simulink model "Formation"  (R2024b)
settings: Solver=ode4  StartTime=0.0  StopTime=50  RelTol=1e-3
libraries: simulink x5
settings Model: Creator=Omar  LastModifiedBy=Omar

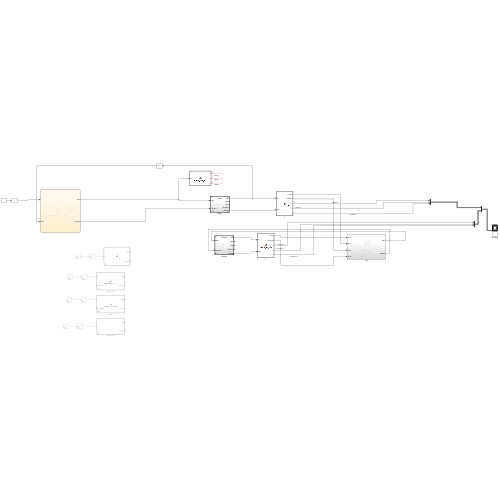
[thumbnail: Simulink's stored preview of the top-level diagram]
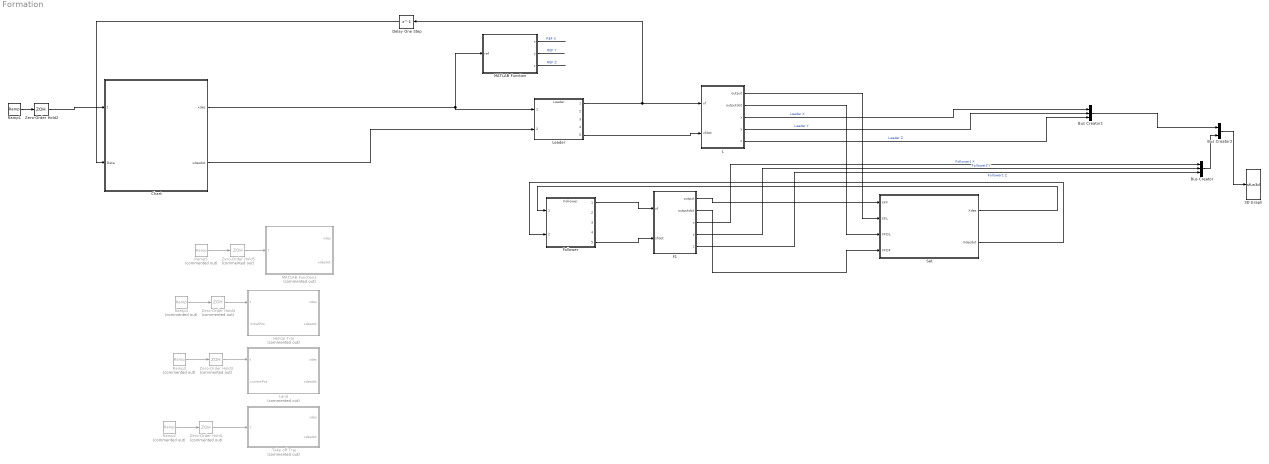
== system Formation ==
  3D Graph : S-Function  LoadFcn=if exist('sfun3d','file'), sfun3d([],[],[],'LoadBlock'); end  FunctionName=sfun3d  Parameters=ax,T,np,cp,gd,ls,mk,mx,hd,tb  SFunctionDeploymentMode=off  EnableBusSupport=off  mask(3D Graph){np=2, ax=[-2 2 -2 2 0 10], mx=1e4, T=0.1, cp=[2 1 3], gd=on, hd=on, tb=off, ls=-, mk=none}
      mask prompts: np "Number of moving points (lines)"; ax "Range: [xmin xmax  ymin ymax zmin zmax]"; mx "Max number of points in each line"; T "Sampling Time"; cp "Camera position (use [0 0 1] for 2D XY view)"; gd "Grid (on|off)"; hd "HeadMarkers (on|off)"; tb "Toolbar (on|off)"; ls "LineStyle"; mk "LineMarker"
      mask help:
      | This block plots the position of several points in the XYZ space. The input contains the coordinates of all the points (x1,y1,z1,x2,y2,z2,...).
      | The number of moving points (lines), the XYZ ranges, sampling time, camera position, and grid (among other things) can be set as mask parameters.
      settings: CopyFcn=if exist('sfun3d','file'), sfun3d([],[],[],'CopyBlock'); end  DeleteFcn=if exist('sfun3d','file'), sfun3d([],[],[],'DeleteBlock'); end  NameChangeFcn=if exist('sfun3d','file'), sfun3d([],[],[],'NameChange'); end
      mask Help:
      | This block plots the position of several points in the XYZ space. The input contains the coordinates of all the points (x1,y1,z1,x2,y2,z2,...).
      | The number of moving points (lines), the XYZ ranges, sampling time, camera position, and grid (among other things) can be set as mask parameters.
      mask TypeOptions ls: - | -- | : | -. | none
      mask TypeOptions mk: none | . | + | o | * | x | square | diamond | v | ^ | > | < | pentagram | hexagram
      mask Display: plot([.05 .95 .95 .05 .05],[.45 .45 .95 .95 .45], 0.5+cos(0:0.1:2*pi)*0.3,0.7+sin(0:0.1:2*pi)*0.2)
  Bus Creator : BusCreator  Inputs=3
  Bus Creator1 : BusCreator  Inputs=3
  Bus Creator2 : BusCreator  Inputs=2
  Chart : Stateflow chart  TreatAsAtomicUnit=on
      settings: PortSchema="{\"entries\":[{\"content\":{\"sides\":[{\"content\":{\"connectorIds\":[\"In1\",\"In2\"]},\"type\":\"ConnectorPlacement.EquallySpacedRectSide\",\"uuid\":\"b3e650a5-816a-4038-bd6f-7a09548ffccf\"},{\"content\":{\"connectorIds\":[\"Out2\",\"Out1\"],\"side\":\"RIGHT\"},\"type\":\"ConnectorPlacement.EquallySpacedRectSide\",\"uuid\":\"881456fa-c96c-4b3e-8437-ce6d3f72eb13\"},{\"content\":{\"side\":\"TOP\"},\"type\":\"ConnectorPlacement.EquallySpacedRectSide\",\"uuid\":\"2026285f-4a20-43d0-8312-bd14694b0db2\"}]},\"type\":\"ConnectorPlacement.EquallySpacedConnector\",\"uuid\":\"eb1cc1af-b444-4b44-9b14-5798d5451655\"}],\"packageUris\":[\"http://schema.mathworks.com/mf0/Connector/R2020b\"],\"version\":\"1.0\"}"
  Delay One Step : Delay  DelayLength=1
  F1 : MATLAB Function  TreatAsAtomicUnit=on
  Follower : ModelReference  ModelNameDialog=Follower.slx  SimulationMode=Normal  ModelReferenceVersion=10.12
  Helical Traj : MATLAB Function  Commented=on  TreatAsAtomicUnit=on
  L : MATLAB Function  TreatAsAtomicUnit=on
  Land : MATLAB Function  Commented=on  TreatAsAtomicUnit=on
  Leader : ModelReference  ModelNameDialog=Leader.slx  SimulationMode=Normal  ModelReferenceVersion=10.10
  MATLAB Function : MATLAB Function  TreatAsAtomicUnit=on
  MATLAB Function1 : MATLAB Function  Commented=on  TreatAsAtomicUnit=on
  Ramp1 : simulink/Sources/Ramp  slope=1  start=0  InitialOutput=0
  Ramp{2..5} (4 alike) : simulink/Sources/Ramp  Commented=on  slope=1  start=0  InitialOutput=0
  Sat : Subsystem
  Take off Traj : MATLAB Function  Commented=on  TreatAsAtomicUnit=on
  Zero-Order Hold{1,3..5} (4 alike) : ZeroOrderHold  Commented=on  SampleTime=0.02
  Zero-Order Hold2 : ZeroOrderHold  SampleTime=0.02
  wires:
  L/3(x) -> Bus Creator1/1  "Leader X"
  L/4(y) -> Bus Creator1/2  "Leader Y"
  L/5(z) -> Bus Creator1/3  "Leader Z"
  F1/4(y) -> Bus Creator/2  "Follower1 Y"
  F1/5(z) -> Bus Creator/3  "Follower1 Z"
  Follower/1 -> F1/1(xf)
  F1/3(x) -> Bus Creator/1  "Follower1 X"
  MATLAB Function/2(y) -> ?  "REF Y"
  MATLAB Function/3(z) -> ?  "REF Z"
  MATLAB Function/1(x) -> ?  "REF X"
  Leader/5 -> L/2(xfdot)
  Follower/5 -> F1/2(xfdot)
  Bus Creator2/1 -> 3D Graph/1
  Bus Creator1/1 -> Bus Creator2/1
  Bus Creator/1 -> Bus Creator2/2
  L/2(outputdot) -> Sat/3(XFDL)
  L/1(output) -> Sat/2(XFL)
  Ramp1/1 -> Zero-Order Hold2/1
  Ramp2/1 -> Zero-Order Hold1/1
  Zero-Order Hold1/1 -> Take off Traj/1(t)
  Ramp3/1 -> Zero-Order Hold3/1
  Zero-Order Hold3/1 -> Land/1(t)
  Zero-Order Hold4/1 -> Helical Traj/1(t)
  Ramp4/1 -> Zero-Order Hold4/1
  Zero-Order Hold2/1 -> Chart/1(t)
  Leader/1 -> Delay One Step/1, L/1(xf)
  Delay One Step/1 -> Chart/2(Data)
  F1/2(outputdot) -> Sat/4(XFDF)
  F1/1(output) -> Sat/1(XFF)
  Ramp5/1 -> Zero-Order Hold5/1
  Zero-Order Hold5/1 -> MATLAB Function1/1(t)
  Chart/2(xdes) -> Leader/1, MATLAB Function/1(ref)
  Chart/1(xdesdot) -> Leader/2
  Sat/2(Xdesdot) -> Follower/2
  Sat/1(Xdes) -> Follower/1

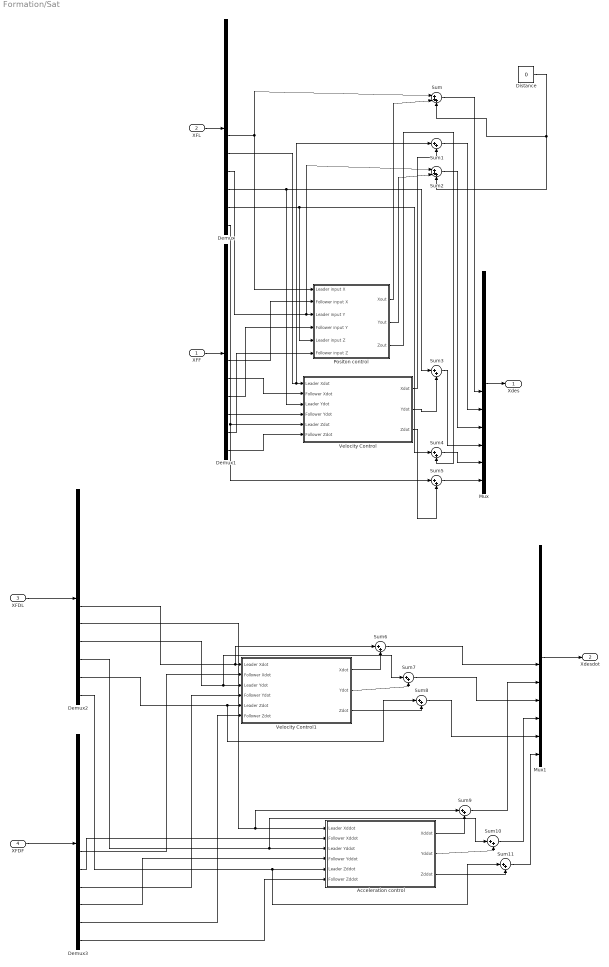
== system Formation/Sat ==
  XFF : Inport
  XFL : Inport  Port=2
  XFDL : Inport  Port=3
  XFDF : Inport  Port=4
  Acceleration control : Subsystem
  Demux{,1..3} (4 alike) : Demux  Outputs=12
  Distance : Constant  Value=0
  Mux : Mux  Inputs=12
  Mux1 : Mux  Inputs=12
  Positon control : Subsystem
  Sum : Sum  Inputs=|+++
  Sum{1,3..11} (10 alike) : Sum  Inputs=|++
  Sum2 : Sum  Inputs=|+++
  Velocity Control : Subsystem
  Velocity Control1 : Subsystem
  Xdes : Outport
  Xdesdot : Outport  Port=2
  wires:
  XFF/1 -> Demux1/1
  XFL/1 -> Demux/1
  Positon control/2(Yout) -> Sum2/2
  Demux/8 -> Sum1/1, Velocity Control/1(Leader Xdot)
  Demux/12 -> Sum5/1, Velocity Control/5(Leader Zdot)
  Demux/7 -> Sum/1, Positon control/1(Leader input X)
  Demux/11 -> Sum4/1, Positon control/5(Leader input Z)
  Demux/10 -> Sum3/1, Velocity Control/3(Leader Ydot)
  Demux/9 -> Sum2/1, Positon control/3(Leader input Y)
  Demux1/11 -> Positon control/6(Follower input Z)
  Demux1/7 -> Positon control/2(Follower input X)
  Demux1/12 -> Velocity Control/6(Follower Zdot)
  Demux1/8 -> Velocity Control/2(Follower Xdot)
  Demux1/9 -> Positon control/4(Follower input Y)
  Demux1/10 -> Velocity Control/4(Follower Ydot)
  Positon control/1(Xout) -> Sum/2
  Positon control/3(Zout) -> Sum4/2
  Velocity Control/1(Xdot) -> Sum1/2
  Velocity Control/2(Ydot) -> Sum3/2
  Velocity Control/3(Zdot) -> Sum5/2
  Sum2/1 -> Mux/9
  Sum/1 -> Mux/7
  Sum3/1 -> Mux/10
  Sum1/1 -> Mux/8
  Sum4/1 -> Mux/11
  Sum5/1 -> Mux/12
  Mux/1 -> Xdes/1
  Mux1/1 -> Xdesdot/1
  Velocity Control1/1(Xdot) -> Sum6/2
  Velocity Control1/2(Ydot) -> Sum7/2
  Velocity Control1/3(Zdot) -> Sum8/2
  XFDL/1 -> Demux2/1
  Demux2/7 -> Sum6/1, Velocity Control1/1(Leader Xdot)
  Demux2/9 -> Sum7/1, Velocity Control1/3(Leader Ydot)
  Demux2/11 -> Sum8/1, Velocity Control1/5(Leader Zdot)
  Demux3/11 -> Velocity Control1/6(Follower Zdot)
  XFDF/1 -> Demux3/1
  Demux3/9 -> Velocity Control1/4(Follower Ydot)
  Demux3/7 -> Velocity Control1/2(Follower Xdot)
  Sum6/1 -> Mux1/7
  Sum7/1 -> Mux1/9
  Sum8/1 -> Mux1/11
  Sum10/1 -> Mux1/10
  Demux2/10 -> Sum10/1, Acceleration control/3(Leader Yddot)
  Sum9/1 -> Mux1/8
  Demux2/8 -> Sum9/1, Acceleration control/1(Leader Xddot)
  Acceleration control/3(Zddot) -> Sum11/2
  Demux3/10 -> Acceleration control/4(Follower Yddot)
  Demux2/12 -> Sum11/1, Acceleration control/5(Leader Zddot)
  Sum11/1 -> Mux1/12
  Demux3/12 -> Acceleration control/6(Follower Zddot)
  Acceleration control/2(Yddot) -> Sum10/2
  Demux3/8 -> Acceleration control/2(Follower Xddot)
  Acceleration control/1(Xddot) -> Sum9/2
  Distance/1 -> Sum/3, Sum2/3

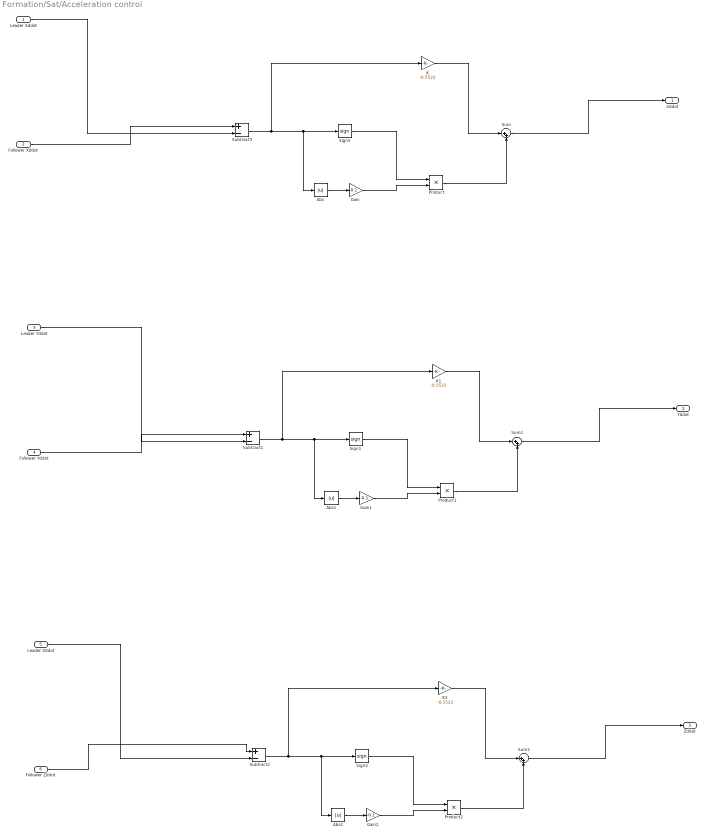
== system Formation/Sat/Acceleration control ==
  Leader Xddot : Inport
  Follower Xddot : Inport  Port=2
  Leader Yddot : Inport  Port=3
  Follower Yddot : Inport  Port=4
  Leader Zddot : Inport  Port=5
  Follower Zddot : Inport  Port=6
  Abs : Abs  SaturateOnIntegerOverflow=off
  Abs1 : Abs  SaturateOnIntegerOverflow=off
  Abs2 : Abs  SaturateOnIntegerOverflow=off
  Gain : Gain  Gain=-0.1
  Gain1 : Gain  Gain=-0.1
  Gain2 : Gain  Gain=-0.1
  K : Gain  Gain=-0.5522
  K1 : Gain  Gain=-0.5522
  K2 : Gain  Gain=-0.5522
  Product : Product
  Product1 : Product
  Product2 : Product
  Sign1 : Signum
  Sign2 : Signum
  Sign5 : Signum
  Subtract1 : Sum  Inputs=+-
  Subtract2 : Sum  Inputs=+-
  Subtract3 : Sum  Inputs=+-
  Sum : Sum  Inputs=|++
  Sum1 : Sum  Inputs=|++
  Sum2 : Sum  Inputs=|++
  Xddot : Outport
  Yddot : Outport  Port=2
  Zddot : Outport  Port=3
  wires:
  Sign5/1 -> Product/1
  Follower Xddot/1 -> Subtract3/1
  Abs/1 -> Gain/1
  Product/1 -> Sum/2
  Gain/1 -> Product/2
  K/1 -> Sum/1
  Subtract3/1 -> K/1, Abs/1, Sign5/1
  Leader Xddot/1 -> Subtract3/2
  Sum/1 -> Xddot/1
  Gain1/1 -> Product1/2
  Product1/1 -> Sum1/2
  Subtract1/1 -> K1/1, Abs1/1, Sign1/1
  K1/1 -> Sum1/1
  Sign1/1 -> Product1/1
  Sum1/1 -> Yddot/1
  Follower Yddot/1 -> Subtract1/1
  Leader Yddot/1 -> Subtract1/2
  Abs1/1 -> Gain1/1
  Sum2/1 -> Zddot/1
  Sign2/1 -> Product2/1
  Leader Zddot/1 -> Subtract2/2
  Subtract2/1 -> K2/1, Abs2/1, Sign2/1
  Follower Zddot/1 -> Subtract2/1
  Gain2/1 -> Product2/2
  K2/1 -> Sum2/1
  Product2/1 -> Sum2/2
  Abs2/1 -> Gain2/1

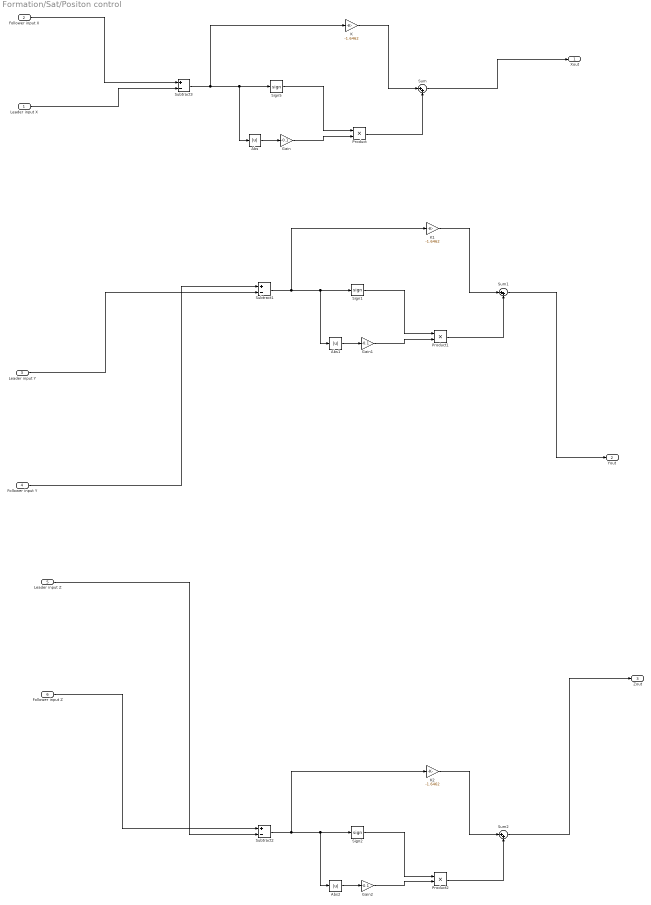
== system Formation/Sat/Positon control ==
  Leader input X : Inport
  Follower input X : Inport  Port=2
  Leader input Y : Inport  Port=3
  Follower input Y : Inport  Port=4
  Leader input Z : Inport  Port=5
  Follower input Z : Inport  Port=6
  Abs : Abs  SaturateOnIntegerOverflow=off
  Abs1 : Abs  SaturateOnIntegerOverflow=off
  Abs2 : Abs  SaturateOnIntegerOverflow=off
  Gain : Gain  Gain=-0.1
  Gain1 : Gain  Gain=-0.1
  Gain2 : Gain  Gain=-0.1
  K : Gain  Gain=-1.6462
  K1 : Gain  Gain=-1.6462
  K2 : Gain  Gain=-1.6462
  Product : Product
  Product1 : Product
  Product2 : Product
  Sign1 : Signum
  Sign2 : Signum
  Sign5 : Signum
  Subtract1 : Sum  Inputs=+-
  Subtract2 : Sum  Inputs=+-
  Subtract3 : Sum  Inputs=+-
  Sum : Sum  Inputs=|++
  Sum1 : Sum  Inputs=|++
  Sum2 : Sum  Inputs=|++
  Xout : Outport
  Yout : Outport  Port=2
  Zout : Outport  Port=3
  wires:
  Subtract3/1 -> K/1, Abs/1, Sign5/1
  Follower input X/1 -> Subtract3/1
  K/1 -> Sum/1
  Product/1 -> Sum/2
  Abs/1 -> Gain/1
  Sign5/1 -> Product/1
  Gain/1 -> Product/2
  Sum/1 -> Xout/1
  Leader input X/1 -> Subtract3/2
  Gain1/1 -> Product1/2
  Sign1/1 -> Product1/1
  Product1/1 -> Sum1/2
  Leader input Y/1 -> Subtract1/2
  Subtract1/1 -> K1/1, Abs1/1, Sign1/1
  Abs1/1 -> Gain1/1
  Follower input Y/1 -> Subtract1/1
  K1/1 -> Sum1/1
  Sum1/1 -> Yout/1
  Sum2/1 -> Zout/1
  Follower input Z/1 -> Subtract2/1
  Product2/1 -> Sum2/2
  Gain2/1 -> Product2/2
  Abs2/1 -> Gain2/1
  Leader input Z/1 -> Subtract2/2
  K2/1 -> Sum2/1
  Subtract2/1 -> K2/1, Abs2/1, Sign2/1
  Sign2/1 -> Product2/1

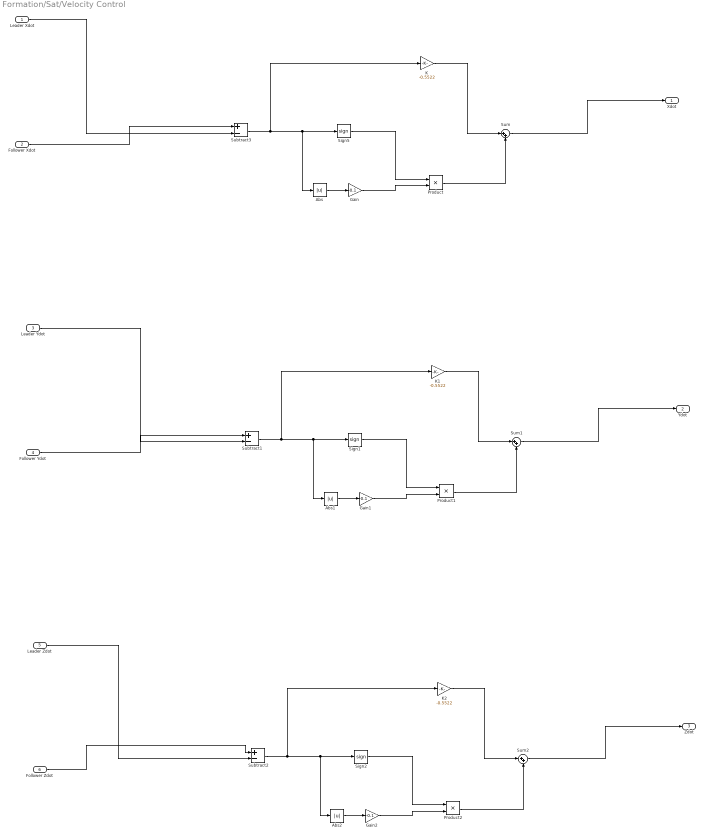
== system Formation/Sat/Velocity Control ==
  Leader Xdot : Inport
  Follower Xdot : Inport  Port=2
  Leader Ydot : Inport  Port=3
  Follower Ydot : Inport  Port=4
  Leader Zdot : Inport  Port=5
  Follower Zdot : Inport  Port=6
  Abs : Abs  SaturateOnIntegerOverflow=off
  Abs1 : Abs  SaturateOnIntegerOverflow=off
  Abs2 : Abs  SaturateOnIntegerOverflow=off
  Gain : Gain  Gain=-0.1
  Gain1 : Gain  Gain=-0.1
  Gain2 : Gain  Gain=-0.1
  K : Gain  Gain=-0.5522
  K1 : Gain  Gain=-0.5522
  K2 : Gain  Gain=-0.5522
  Product : Product
  Product1 : Product
  Product2 : Product
  Sign1 : Signum
  Sign2 : Signum
  Sign5 : Signum
  Subtract1 : Sum  Inputs=+-
  Subtract2 : Sum  Inputs=+-
  Subtract3 : Sum  Inputs=+-
  Sum : Sum  Inputs=|++
  Sum1 : Sum  Inputs=|++
  Sum2 : Sum  Inputs=|++
  Xdot : Outport
  Ydot : Outport  Port=2
  Zdot : Outport  Port=3
  wires:
  Sign5/1 -> Product/1
  Follower Xdot/1 -> Subtract3/1
  Abs/1 -> Gain/1
  Product/1 -> Sum/2
  Gain/1 -> Product/2
  K/1 -> Sum/1
  Subtract3/1 -> K/1, Abs/1, Sign5/1
  Leader Xdot/1 -> Subtract3/2
  Sum/1 -> Xdot/1
  Gain1/1 -> Product1/2
  Product1/1 -> Sum1/2
  Subtract1/1 -> K1/1, Abs1/1, Sign1/1
  K1/1 -> Sum1/1
  Sign1/1 -> Product1/1
  Sum1/1 -> Ydot/1
  Follower Ydot/1 -> Subtract1/1
  Leader Ydot/1 -> Subtract1/2
  Abs1/1 -> Gain1/1
  Sum2/1 -> Zdot/1
  Sign2/1 -> Product2/1
  Leader Zdot/1 -> Subtract2/2
  Subtract2/1 -> K2/1, Abs2/1, Sign2/1
  Follower Zdot/1 -> Subtract2/1
  Gain2/1 -> Product2/2
  K2/1 -> Sum2/1
  Product2/1 -> Sum2/2
  Abs2/1 -> Gain2/1

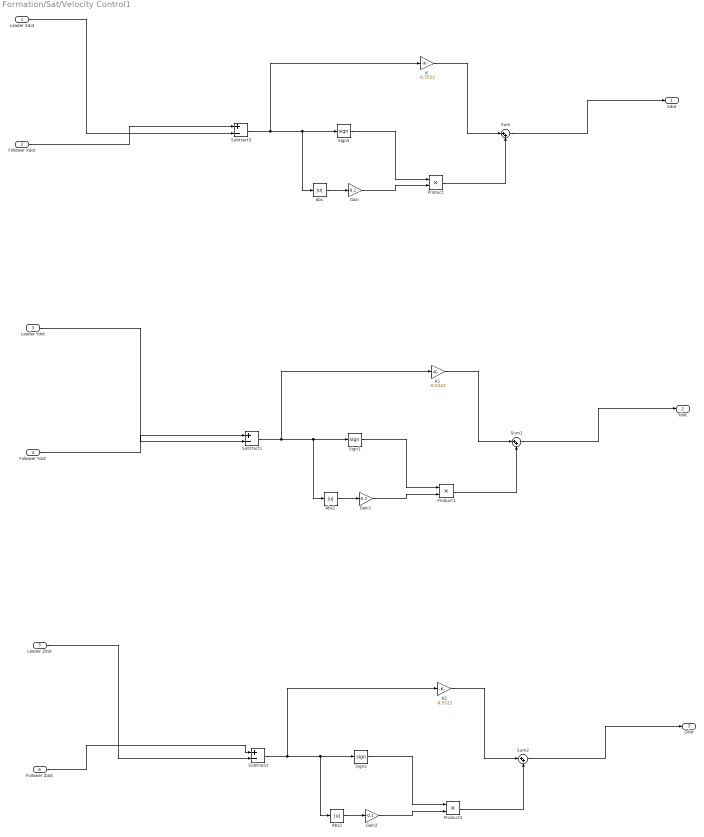
== system Formation/Sat/Velocity Control1 ==
  Leader Xdot : Inport
  Follower Xdot : Inport  Port=2
  Leader Ydot : Inport  Port=3
  Follower Ydot : Inport  Port=4
  Leader Zdot : Inport  Port=5
  Follower Zdot : Inport  Port=6
  Abs : Abs  SaturateOnIntegerOverflow=off
  Abs1 : Abs  SaturateOnIntegerOverflow=off
  Abs2 : Abs  SaturateOnIntegerOverflow=off
  Gain : Gain  Gain=-0.1
  Gain1 : Gain  Gain=-0.1
  Gain2 : Gain  Gain=-0.1
  K : Gain  Gain=-0.5522
  K1 : Gain  Gain=-0.5522
  K2 : Gain  Gain=-0.5522
  Product : Product
  Product1 : Product
  Product2 : Product
  Sign1 : Signum
  Sign2 : Signum
  Sign5 : Signum
  Subtract1 : Sum  Inputs=+-
  Subtract2 : Sum  Inputs=+-
  Subtract3 : Sum  Inputs=+-
  Sum : Sum  Inputs=|++
  Sum1 : Sum  Inputs=|++
  Sum2 : Sum  Inputs=|++
  Xdot : Outport
  Ydot : Outport  Port=2
  Zdot : Outport  Port=3
  wires:
  Sign5/1 -> Product/1
  Follower Xdot/1 -> Subtract3/1
  Abs/1 -> Gain/1
  Product/1 -> Sum/2
  Gain/1 -> Product/2
  K/1 -> Sum/1
  Subtract3/1 -> K/1, Abs/1, Sign5/1
  Leader Xdot/1 -> Subtract3/2
  Sum/1 -> Xdot/1
  Gain1/1 -> Product1/2
  Product1/1 -> Sum1/2
  Subtract1/1 -> K1/1, Abs1/1, Sign1/1
  K1/1 -> Sum1/1
  Sign1/1 -> Product1/1
  Sum1/1 -> Ydot/1
  Follower Ydot/1 -> Subtract1/1
  Leader Ydot/1 -> Subtract1/2
  Abs1/1 -> Gain1/1
  Sum2/1 -> Zdot/1
  Sign2/1 -> Product2/1
  Leader Zdot/1 -> Subtract2/2
  Subtract2/1 -> K2/1, Abs2/1, Sign2/1
  Follower Zdot/1 -> Subtract2/1
  Gain2/1 -> Product2/2
  K2/1 -> Sum2/1
  Product2/1 -> Sum2/2
  Abs2/1 -> Gain2/1

== matlab function Formation/Land ==
  data: t input; xdes output; xdesdot output; currentPos input
function [xdes, xdesdot] = TrajectoryPlanner(t,currentPos)

    % Define the target z position
    z_target = 0.0;   % Target position (ground level)
    
    % Define the landing time (e.g., 10 seconds to land)
    landing_time = 10.0; 

    % Get the current z position from the currentPos input
    z_current = currentPos(11);

    % Linearly decrease z until it reaches 0
    z = max(z_target, z_current - (z_current / landing_time) * t);  % Decrease z over time
    zdot = (z > z_target) * (-z_current / landing_time);  % Vertical velocity is negative until it reaches 0, then 0

    % Define the desired state: [phi p theta q psi r x xdot y ydot z zdot]
    xdes = [0 0 0 0 0 0 currentPos(7) 0 currentPos(9) 0 z zdot]';
    xdesdot = [0 0 0 0 0 0 0 0 0 0 zdot 0]';

end

== matlab function Formation/MATLAB Function1 ==
  data: xdes output; xdesdot output; t input
function [xdes, xdesdot] = StayAtZ1(t)
    % Inputs:
    % t - Current time
    
    % Define the target z position
    z_target = 1.0;  % Target z position (1 meter high)
    
    % Define the speed in x and y direction (no movement in x and y)
    speed_x = 0.0;  % No movement in x direction
    speed_y = 0.0;  % No movement in y direction

    % Define the takeoff time (e.g., 5 seconds to reach z = 1)
    takeoff_time = 5.0;
    
    % Linearly increase z until it reaches the target height (1 meter)
    z = min(z_target, 0.2 * t);  % z increases at a rate of 0.2 meters per second

    % Once z reaches 1, the drone stays at z = 1 and does not move
    if t > takeoff_time
        z = z_target;  % Stay at z = 1 after takeoff
    end

    % Set x and y to 0 as the drone stays at (0, 0)
    x = 0;
    y = 0;

    % Compute velocities for x, y, and z
    xdot = 0;  % No movement in x-direction
    ydot = 0;  % No movement in y-direction
    zdot = (z < z_target) * 0.2;  % Vertical velocity (0.2 m/s until z = 1)

    % Define the desired state: [phi p theta q psi r x xdot y ydot z zdot]
    xdes = [0 0 0 0 0 0 x xdot y ydot z zdot]';
    
    % Define the rate of change of the desired state
    xdesdot = [0 0 0 0 0 0 xdot 0 ydot 0 zdot 0]';
end

== matlab function Formation/F1 ==
  data: output output; outputdot output; x output; xf input; y output; z output; xfdot input
function [output,outputdot,x,y,z]= remove_last_two(xf,xfdot)
    % Remove the last two elements of a 16x1 vector
    outputdot= xfdot(1:end-4);
    output = xf(1:end-4);
    x = output(7);
    y = output(9);
    z = output(11);
end

== matlab function Formation/L ==
  data: output output; outputdot output; x output; xf input; y output; z output; xfdot input
function [output,outputdot,x,y,z]= remove_last_two(xf,xfdot)
    % Remove the last two elements of a 16x1 vector
    outputdot= xfdot(1:end-4);
    output = xf(1:end-4);
    x = output(7);
    y = output(9);
    z = output(11);
end

== matlab function Formation/MATLAB Function ==
  data: x output; ref input; y output; z output
function [x,y,z]= remove_last_two(ref)
    x = ref(7);
    y = ref(9);
    z = ref(11);
end

== matlab function Formation/Helical Traj ==
  data: xdes output; xdesdot output; t input; initialPos input
function [xdes, xdesdot] = TrajectoryPlanner(t, initialPos)
persistent savedInitialPos; % Persistent variable to store the initial position

    %If it's the first call, save the initial position
    if isempty(savedInitialPos)
        savedInitialPos = initialPos;
    end
    % Fixed omega and Vz %
    % Define the main parameters of the helix
    % w = 3.0;
    % Vz = 1.0;
    % r = 1.0;
    
    %xdes = [phi p theta q psi r x xdot y ydot z zdot]
    xdes = [0 0 0 0 0 0 savedInitialPos(7)+cos(t) -sin(t) savedInitialPos(9)+sin(t) cos(t) savedInitialPos(11)+0.5*t 0.5]';
    xdesdot = [0 0 0 0 0 0 -sin(t) -cos(t) cos(t) -sin(t) 0.5 0]';

end

== matlab function Formation/Take off Traj ==
  data: t input; xdes output; xdesdot output
function [xdes, xdesdot] = TrajectoryPlanner(t)


        % Define the desired z position as it approaches z = 1
        z = min(1.0, 0.2 * t); % Linearly increase z until it reaches 1.0, slower than before
        zdot = (z < 1.0) * 0.2; % z velocity is 0.2 until z reaches 1.0, then it is 0

        % xdes = [phi p theta q psi r x xdot y ydot z zdot]
        xdes = [0 0 0 0 0 0 0 0 0 0 z zdot]';
        xdesdot = [0 0 0 0 0 0 0 0 0 0 zdot 0]';
        
end

== stateflow chart Formation/Chart ==
  state Takeoff
    [xdes, xdesdot,hd] = Takeoff(t,Data);
  state Off
    if done == true
    [xdes,xdesdot]=Staystill(t,Data)
    end
  state circle
    [xdes, xdesdot,comp] = circle(t,Data);
  (default) -> Off : {done = false}
  Off -> Takeoff : [done == false]
  Takeoff -> circle : [hd==true]
  circle -> Off : [comp == true]{done =true}
  data: t input; xdesdot output; xdes output; done local; Data input; hd local; comp local
